simulink model "free_response"  (R2024b)
settings: Solver=VariableStepAuto  StartTime=0.0  StopTime=10.0  RelTol=1e-3
values from neighbouring files (symbols this model uses):
  A = output{1}    [task1.m]
  B = output{2}    [task1.m]
  C = output{3}    [task1.m]
  K = K_bar_sol*T    [task1.m]
  x_0 = output{5}    [task1.m]
settings Model: Creator=KevinNuo  LastModifiedBy=KevinNuo

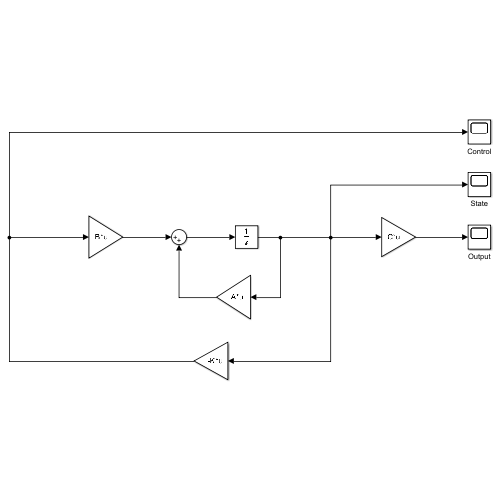
[thumbnail: Simulink's stored preview of the top-level diagram]
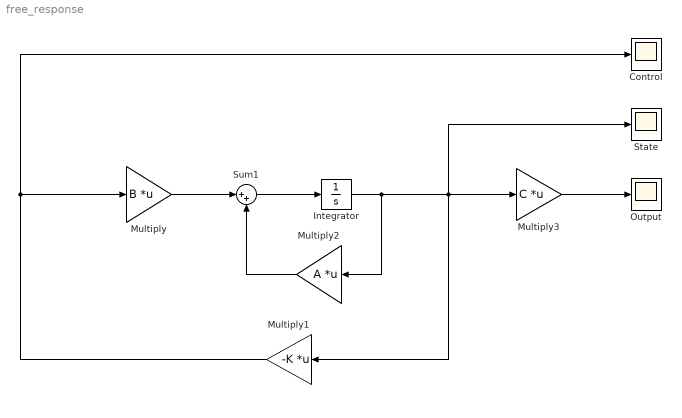
== system free_response ==
  Control : Scope
  Integrator : Integrator  InitialCondition=x_0
  Multiply : Gain  Gain=B  Multiplication=Matrix(K*u)
  Multiply1 : Gain  Gain=-K  Multiplication=Matrix(K*u)
  Multiply2 : Gain  Gain=A  Multiplication=Matrix(K*u)
  Multiply3 : Gain  Gain=C  Multiplication=Matrix(K*u)
  Output : Scope
  State : Scope
  Sum1 : Sum  Inputs=|++
  wires:
  Multiply/1 -> Sum1/1
  Sum1/1 -> Integrator/1
  Integrator/1 -> Multiply2/1, State/1, Multiply1/1, Multiply3/1
  Multiply2/1 -> Sum1/2
  Multiply3/1 -> Output/1
  Multiply1/1 -> Control/1, Multiply/1
